simulink library "powerlib_models"  (Simulink 6.0)
settings: Solver=ode45  SolverMode=SingleTasking  StartTime=0.0  StopTime=10.0  RelTol=1e-3
values from neighbouring files (symbols this model uses):
  Ts = get(handles.edit1,'string')    [powergui.m]
undefined symbols (not defined in the file or in its folder): A, a0, a1, a2, a3, a4, a5, Ac, Amplitude, Amplitudes, B, BaseCurrent, BaseFlux, Bc, C, Capacitance, Cc, Columns, ConnectionType, Cs, ctrl, current, Current, damp, Dc, Dd, DiscIntNeverNeededParam, dref, dwo, exc, excAxis, F, Flux, fnom, Frequency, FreqVps, Gain1, gate, GH, GHd, GI, GId, GL, GLd, H, HarmonicGeneration, HT, hyd, I1_init, ib, ib2, Id1o, Inductance, InitialFlux, InitialSlope, io, Iq1o, isfinite, j, J ... (+138)
libraries: powerlib_models x32, powerlib_extras x4
(part 7 of 11)

== system powerlib_models/Discrete/3_Phase_Prog_Source/Harmonic A generation ==
  Enable : Inport  Port=1  LatchInput=off
  Gain2 : Gain  Gain=2*pi*n_Harmo  SaturateOnIntegerOverflow=on
  Gain3 : Gain  Gain=pi/180  SaturateOnIntegerOverflow=on
  Multiport Switch : MultiPortSwitch  Inputs=3  InputSameDT=on
  Negative-sequence : Constant  Value=[0 2*pi/3 -2*pi/3]
  Phase_Harmo : Constant  Value=Phase_Harmo
  Phase_Harmo1 : Constant  Value=Mag_Harmo
  Phase_Harmo2 : Constant  Value=Seq_Harmo
  Positive-sequence : Constant  Value=[0 -2*pi/3 2*pi/3]
  Product : Product  SaturateOnIntegerOverflow=on  InputSameDT=on
  Product1 : Product  Inputs=3  SaturateOnIntegerOverflow=on  InputSameDT=on
  Sum : Sum  Inputs=+++  SaturateOnIntegerOverflow=on  InputSameDT=on
  Sum1 : Sum  SaturateOnIntegerOverflow=on  InputSameDT=on
  Trigonometric Function1 : Trigonometry
  Zero-sequence : Constant  Value=[0 0 0]
  t : DigitalClock  SampleTime=Ts
  valp_nom1 : Constant  Value=Freq_Vps
  valp_nom2 : Constant
  HarmoA : Outport
  wires:
  Gain3/1 -> Sum/2
  Phase_Harmo/1 -> Gain3/1
  Enable/1 -> Product1/1
  valp_nom2/1 -> Sum1/2
  Phase_Harmo2/1 -> Sum1/1
  Sum1/1 -> Multiport Switch/1
  Phase_Harmo1/1 -> Product1/2
  Product1/1 -> HarmoA/1
  Trigonometric Function1/1 -> Product1/3
  Product/1 -> Sum/1
  t/1 -> Product/1
  Gain2/1 -> Product/2
  valp_nom1/1 -> Gain2/1
  Negative-sequence/1 -> Multiport Switch/4
  Positive-sequence/1 -> Multiport Switch/3
  Zero-sequence/1 -> Multiport Switch/2
  Multiport Switch/1 -> Sum/3
  Sum/1 -> Trigonometric Function1/1

== system powerlib_models/Discrete/3_Phase_Prog_Source/Harmonic B generation ==
  Enable : Inport  Port=1  LatchInput=off
  Gain2 : Gain  Gain=2*pi*n_Harmo  SaturateOnIntegerOverflow=on
  Gain3 : Gain  Gain=pi/180  SaturateOnIntegerOverflow=on
  Multiport Switch : MultiPortSwitch  Inputs=3  InputSameDT=on
  Negative-sequence : Constant  Value=[0 2*pi/3 -2*pi/3]
  Phase_Harmo : Constant  Value=Phase_Harmo
  Phase_Harmo1 : Constant  Value=Mag_Harmo
  Phase_Harmo2 : Constant  Value=Seq_Harmo
  Positive-sequence : Constant  Value=[0 -2*pi/3 2*pi/3]
  Product : Product  SaturateOnIntegerOverflow=on  InputSameDT=on
  Product1 : Product  Inputs=3  SaturateOnIntegerOverflow=on  InputSameDT=on
  Sum : Sum  Inputs=+++  SaturateOnIntegerOverflow=on  InputSameDT=on
  Sum1 : Sum  SaturateOnIntegerOverflow=on  InputSameDT=on
  Trigonometric Function1 : Trigonometry
  Zero-sequence : Constant  Value=[0 0 0]
  t : DigitalClock  SampleTime=Ts
  valp_nom1 : Constant  Value=Freq_Vps
  valp_nom2 : Constant
  HarmoB : Outport
  wires:
  Gain3/1 -> Sum/2
  Phase_Harmo/1 -> Gain3/1
  Sum/1 -> Trigonometric Function1/1
  Multiport Switch/1 -> Sum/3
  Zero-sequence/1 -> Multiport Switch/2
  Positive-sequence/1 -> Multiport Switch/3
  Negative-sequence/1 -> Multiport Switch/4
  valp_nom1/1 -> Gain2/1
  Gain2/1 -> Product/2
  t/1 -> Product/1
  Product/1 -> Sum/1
  Trigonometric Function1/1 -> Product1/3
  Product1/1 -> HarmoB/1
  Phase_Harmo1/1 -> Product1/2
  Sum1/1 -> Multiport Switch/1
  Phase_Harmo2/1 -> Sum1/1
  valp_nom2/1 -> Sum1/2
  Enable/1 -> Product1/1

== system powerlib_models/Discrete/3_Phase_Prog_Source/Timer ==
  Clock : Clock
  Look-Up Table : Lookup  DialogController=Simulink.DDGSource  InputValues=tv  OutputValues=opv  SaturateOnIntegerOverflow=on
  Out : Outport
  wires:
  Look-Up Table/1 -> Out/1
  Clock/1 -> Look-Up Table/1

== system powerlib_models/Discrete/3_Phase_Prog_Source/Variation SubSystem ==
  VariationType : Inport  Port=1  LatchInput=off
  Constant : Constant  Value=2
  Constant1 : Constant  Value=0
  Constant2 : Constant
  Constant3 : Constant
  Constant4 : Constant  Value=0
  Constant5 : Constant  Value=0
  Data Type  Conversion1 : DataTypeConversion  OutDataTypeMode=boolean  SaturateOnIntegerOverflow=on  RndMeth=Zero
  Data Type  Conversion2 : DataTypeConversion  Orientation=up  OutDataTypeMode=boolean  SaturateOnIntegerOverflow=on  RndMeth=Zero
  Discrete-Time Integrator1 : DiscreteIntegrator  SampleTime=Ts  ICPrevOutput=DiscIntNeverNeededParam  ICPrevScaledInput=DiscIntNeverNeededParam
  Gain1 : Gain  Gain=2*pi  SaturateOnIntegerOverflow=on
  Logical Operator : Logic
  Logical Operator1 : Logic  Orientation=up  Operator=NOT
  Multiport Switch1 : MultiPortSwitch  InputSameDT=on
  Product : Product  SaturateOnIntegerOverflow=on  InputSameDT=on
  Product1 : Product  SaturateOnIntegerOverflow=on  InputSameDT=on
  Product2 : Product  SaturateOnIntegerOverflow=on  InputSameDT=on
  Relational Operator : RelationalOperator  Operator===  InputSameDT=on
  Relational Operator1 : RelationalOperator  Operator===  InputSameDT=on
  Step : Step  Time=Ton_Variation  SampleTime=Ts
  Step1 : Step  Time=Toff_Variation  Before=1  After=0  SampleTime=Ts
  Switch{,1..3} (4 alike) : Switch  Threshold=0.5  InputSameDT=on
  Trigonometric Function1 : Trigonometry
  Unit Delay : UnitDelay  Orientation=left  SampleTime=Ts
  valp_nom6 : Constant  Value=VariationStep
  valp_nom7 : Constant  Value=VariationRate
  valp_nom8 : Constant  Value=VariationMag
  valp_nom9 : Constant  Value=VariationFreq
  Value : Outport
  wires:
  Data Type  Conversion1/1 -> Logical Operator/2
  Constant5/1 -> Multiport Switch1/5
  Logical Operator1/1 -> Logical Operator/1
  Logical Operator/1 -> Switch3/2
  Step1/1 -> Switch2/2, Data Type  Conversion2/1  "Toff"
  Constant3/1 -> Relational Operator1/2
  Switch3/1 -> Value/1
  Switch2/1 -> Switch3/3, Unit Delay/1
  Constant1/1 -> Switch3/1
  Unit Delay/1 -> Switch2/3
  Multiport Switch1/1 -> Switch2/1
  Step/1 -> Product2/2, Switch/2  "Ton"
  VariationType/1 -> Relational Operator/1, Relational Operator1/1, Multiport Switch1/1
  Discrete-Time Integrator1/1 -> Multiport Switch1/3, Product1/1  "Ramp"
  Product2/1 -> Multiport Switch1/2  "Step"
  valp_nom6/1 -> Product2/1
  Relational Operator/1 -> Switch1/2
  Switch/1 -> Discrete-Time Integrator1/1
  Constant/1 -> Relational Operator/2
  Switch1/1 -> Switch/1
  Constant4/1 -> Switch/3
  Constant2/1 -> Switch1/3
  valp_nom7/1 -> Switch1/1
  Product/1 -> Multiport Switch1/4  "Mod"
  Product1/1 -> Trigonometric Function1/1
  Gain1/1 -> Product1/2
  valp_nom9/1 -> Gain1/1
  valp_nom8/1 -> Product/1
  Trigonometric Function1/1 -> Product/2
  Data Type  Conversion2/1 -> Logical Operator1/1
  Relational Operator1/1 -> Data Type  Conversion1/1

== system powerlib_models/Discrete/Dynamic_Load/Discrete 3-phase PLL ==
  note: Pierre Giroux, Gilbert Sybille
      | Power System Laboratory, IREQ
      | Hydro-Quebec
  note: Discrete 3-phase PLL
  note: link disabled
  note: link disabled
  note: link disabled
  note: link disabled
  note: link broken
  Vab_bc (pu) : Inport  Port=1  PortDimensions=2  LatchInput=off
  Constant4 : Constant  Value=2*pi
  Discrete PI Controller : Subsystem  AncestorBlock=|  mask(Discrete PI Controller){Kp=Kp, Ki=Ki, Par_Limits=2*pi*Finit*[1.25 0.75], Init=2*pi*Finit, Ts=Ts}
      | powerlib_extras/Discrete 
      | Control Blocks/Discrete
      | PI Controller
      mask prompts: Kp "Proportional gain (Kp):"; Ki "Integral gain (Ki):"; Par_Limits "Output limits: [ Upper   Lower ]"; Init "Output initial value:"; Ts "Sample time:"
      mask help: This block implements a discrete PI controller.
      mask init:
      | UpperLimit=Par_Limits(1);
      | LowerLimit=Par_Limits(2);
      mask Display: disp('PI');
  Discrete Rate Limiter : Subsystem  AncestorBlock=|  mask{R=10, F=-10, Vinit=Finit, Ts=Ts}
      | powerlib_extras/Discrete 
      | Control Blocks/Discrete
      | Rate Limiter
      mask prompts: R "Rising slew rate:"; F "Falling slew rate:"; Vinit "Initial input:"; Ts "Sample time:"
      mask help: DISCRETE BLOCK : Limit rising and falling rates of signal
      mask init:
      | UpperLimit=R*Ts;
      | LowerLimit=F*Ts;
      mask Display: disp('Discrete\nRate\nLimiter')
  Discrete Variable Frequency Mean value : Subsystem  AncestorBlock=|  mask(Discrete Variable-Frequency Mean Value){Finit=Finit, Fmin=45, Vinit=0, Ts=Ts}
      | powerlib_extras/Discrete
      | Measurements/Discrete
      | Variable Frequency
      | Mean value
      mask prompts: Finit "Initial frequency (Hz):"; Fmin "Minimum frequency (Hz):"; Vinit "Initial input (DC component):"; Ts "Sample time:"
      mask help:
      | This discrete block computes the mean value of the input signal (port In) over a running window of one cycle of a specified frequency (port Freq).
      |
      | For the first cycle of simulation (specified by the parameter "Initial frequency"), the ouput is held to the value of the  "Initial input" parameter.
      |
      | The value of the parameter "Minimum frequency" is used to determine the buffer size of the "Variable Transport Delay" block found inside this subsystem.
      mask init:
      | MaxDelay=1/Fmin+Ts;
  Discrete  2nd-Order Filter : Subsystem  AncestorBlock=|  mask(Discrete 2nd-Order Filter){FilterType=Lowpass, Fo=25, Zeta=0.707, Ts=Ts, Initialize=on, Vac_Init=[0 0 Finit], Vdc_Init=Finit, PlotResponse=off, param1=[1 500 0.1]}
      | powerlib_extras/Discrete 
      | Control Blocks/Discrete 
      | 2nd-Order
      | Filter
      mask prompts: FilterType "Filter Type:"; Fo "Cut-off frequency (Hz):"; Zeta "Damping factor Zeta ( Q = 1 / (2*Zeta) ):"; Ts "Sample time:"; Initialize "Initialize filter states"; Vac_Init "AC initial input: [ Mag  Phase(degrees)  Freq(Hz) ]"; Vdc_Init "DC Initial input:"; PlotResponse "Plot filter response"; param1 "Frequency range(Hz) : [Start  End  Inc.]"
      mask init:
      | Wo=2*pi*Fo;
      | str=sprintf(' Fo=%iHz\n\n',Fo);
      | switch FilterType
      | case 1, % Lowpass
      |        X=[0 1 2 3 4];
      |        Y=[-2 -2 -3 -4 -4];
      |        n2=0;n1=0;n0=Wo*Wo;
      |        d2=1;d1=2*Zeta*Wo;d0=Wo*Wo;
      |  case 2,   % Highpass
      |        X=[0 1 2 3 4];
      |        Y=[-4 -4 -3 -2 -2];
      |        n2=1;n1=0;n0=0;
      |        d2=1;d1=2*Zeta*Wo;d0=Wo*Wo;
      |     case 3,   % Bandpass
      |        X=[0 1 2 3 4 5 ];
      |        Y=[-3 -3 -2 -2 -3 -3];
      |        n2=0;n1=2*Zeta*Wo;n0=0;
      |        d2=1;d1=2*Zeta*Wo;d0=Wo*Wo;
      |     case 4,  %Bandstop (Notch)
      |        X=[0 1 2 3 4 5 ];
      |        Y=[-2 -2 -3 -3 -2 -2];
      |        n2=1;n1=0;n0=Wo*Wo;
      |        d2=1;d1=2*Zeta*Wo;d0=Wo*Wo;
      |     end
      | %
      | numc=[n2 n1 n0];
      | denc=[d2 d1 d0];
      | [Ac,Bc,Cc,Dc]=tf2ss(numc,denc);
      | %
      | %  Conversion to discrete transfer function
      | nstates = size(Ac,1);
      | invexp = inv(eye(nstates) - (Ts/2)*Ac);
      | Ad = invexp*(eye(nstates) + (Ts/2)*Ac);
      | Bd = invexp*Bc;
      | Cd = Cc*invexp*Ts;
      | Dd = Cc*invexp*Bc*(Ts/2) + Dc;
      | %
      | if Initialize==1  % Compute initial conditions on states
      | u1=Vac_Init(1)*exp(j*Vac_Init(2)*pi/180);
      | u2=Vdc_Init*exp(j*90*pi/180);
      | u=u1+u2;
      | u0=imag(u); % input at  t=0;
      | I=eye(size(Ac));
      | sI1=I*j*(2*pi*Vac_Init(3));
      | sI2=I*j*0;
      | x=inv(sI1-Ac)*Bc*u1 + inv(sI2-Ac)*Bc*u2;
      | x0c=imag(x);
      | x0d=(I-Ac*Ts/2)*x0c/Ts - Bc/2*u0;
      | else
      | x0d=0;
      | end
      | %
      | if PlotResponse==1 % Plot frequency and step response
      | figure(1)
      | sys=ss(Ad,Bd,Cd,Dd,Ts);
      | f=param1(1):param1(3):param1(2);
      | w=2*pi*f;
      | [mag phase]=bode(sys,w);
      | subplot(2,1,1)
      | plot(f,squeeze(mag))
      | title('Magnitude')
      | grid
      | subplot(2,1,2)
      | plot(f,squeeze(phase))
      | title('Phase (degrees)')
      | xlabel('Hz')
      | grid
      | figure(2)
      | step(sys)
      | end
      mask StyleString: popup(Lowpass|Highpass|Bandpass|Bandstop (Notch)),edit,edit,edit,checkbox,edit,edit,checkbox,edit
      mask CallbackString: ||||p5=get_param(gcb,'Initialize');if strcmp(p5,'on');visible={'on','on','on','on','on','on','on','on',get_param(gcb,'PlotResponse')};else;visible={'on','on','on','on','on','off','off','on',get_param(gcb,'PlotResponse')};end;set_param(gcb,'MaskVisibilities',visible)|||p8=get_param(gcb,'PlotResponse');if strcmp(p8,'on');visible={'on','on','on','on','on',get_param(gcb,'Initialize'),get_param(gcb,'Initialize'),'on','on'};else;visible={'on','on','on','on','on',get_param(gcb,'Initialize'),get_param(gcb,'Initialize'),'on','off'};end;set_param(gcb,'MaskVisibilities',visible)|
      mask Display:
      | plot(X,Y);
      | disp(str);
  Discrete-Time Integrator : DiscreteIntegrator  InitialCondition=Phase_Init*pi/180  SampleTime=Ts  ICPrevOutput=DiscIntNeverNeededParam  ICPrevScaledInput=DiscIntNeverNeededParam
  Gain10 : Gain  Gain=1/2/pi  SaturateOnIntegerOverflow=on
  Math Function : Math  Operator=mod  SaturateOnIntegerOverflow=on
  Mux2 : Mux  Inputs=2
  Trigonometric Function : Trigonometry
  Trigonometric Function2 : Trigonometry  Operator=cos
  Unit Delay : UnitDelay  X0=Finit  SampleTime=Ts
  abc_to_dq1 : Subsystem
  Freq : Outport
  Vd : Outport  Port=2
  Vq : Outport  Port=3
  sin_cos : Outport  Port=4
  wires:
  Discrete  2nd-Order Filter/1(Out) -> Unit Delay/1
  Unit Delay/1 -> Discrete Variable Frequency Mean value/1(Freq), Freq/1
  Discrete Rate Limiter/1(Out) -> Discrete  2nd-Order Filter/1(In)
  Gain10/1 -> Discrete Rate Limiter/1(In)
  Discrete PI Controller/1(Out) -> Gain10/1, Discrete-Time Integrator/1  "W"
  Mux2/1 -> sin_cos/1, abc_to_dq1/2(sin_cos)
  Trigonometric Function2/1 -> Mux2/2
  Trigonometric Function/1 -> Mux2/1
  Math Function/1 -> Trigonometric Function2/1, Trigonometric Function/1
  Discrete-Time Integrator/1 -> Math Function/1
  Constant4/1 -> Math Function/2
  abc_to_dq1/2(vq) -> Discrete Variable Frequency Mean value/2(In), Vq/1  "Vq"
  Vab_bc (pu)/1 -> abc_to_dq1/1(Vab_bc)
  Discrete Variable Frequency Mean value/1(Mean) -> Discrete PI Controller/1(Error)
  abc_to_dq1/1(vd) -> Vd/1

== system powerlib_models/Discrete/Dynamic_Load/Positive Sequence  current ==
  note: kp=Vmin^(np-2)/Vo^np
      | kq=Vmin^(nq-2)/Vo^nq
  note: V<Vmin
      | Constant impedance load :
      |  P=Po*kp*V^2
      | Q=Qo*kq*V^2
  note: V>Vmin :
      |
      |    P=Po*(V/Vo)^np
      |    Q=Qo*(V/Vo)^np
  note: I1= (S/V1)'
  note: link disabled
  note: link disabled
  V1(pu) : Inport  Port=1  PortDimensions=1  LatchInput=off
  S_ext : Inport  Port=2  PortDimensions=1  LatchInput=off
  Complex to Magnitude-Angle : ComplexToMagnitudeAngle  Output=Magnitude
  Complex to Real-Imag1 : ComplexToRealImag
  Conj1 : Math  Operator=conj  SaturateOnIntegerOverflow=on
  Math Function : Math  Operator=square  SaturateOnIntegerOverflow=on
  Mux1 : Mux  Inputs=3
  Mux2 : Mux  Inputs=2
  Mux3 : Mux  Inputs=2
  P0/ (Vo^np) : Gain  Gain=P0/(Mag_V0^np)  SaturateOnIntegerOverflow=on
  PQ_ext : Constant  Value=PQext
  Product : Product  Inputs=/*  SaturateOnIntegerOverflow=on  InputSameDT=on
  Q0/(Vo^nq) : Gain  Gain=Q0/(Mag_V0^nq)  SaturateOnIntegerOverflow=on
  Real-Imag to Complex : RealImagToComplex
  Switch1 : Switch  Threshold=0.5  InputSameDT=on
  Switch3 : Switch  Threshold=Vmin  InputSameDT=on
  Switch4 : Switch  Threshold=Vmin  InputSameDT=on
  TF_P : Subsystem  AncestorBlock=|  mask(Discrete Lead-Lag Controller){T1=Tp1, T2=Tp2, V_Init=P0, Ts=Ts}
      | powerlib_extras/Discrete 
      | Control Blocks/Discrete
      | Lead-Lag
      mask prompts: T1 "Time constant T1 (s):"; T2 "Time constant T2 (s):"; V_Init "Initial input and output:"; Ts "Sample time (s):"
      mask help:
      | This block implements a discrete lead-lag controller:
      |
      |          1+T1s
      | H(s)= ------
      |          1+T2s
      |
      | States are initialized according to initial input anf output value so that simulation starts in steady state.
      mask init: same as powerlib_models/Discrete/Excitation_System/Lead Lag Compensator tc.s+1 / tb.s+1
      mask Display: disp('1+T1s\n---\n1+T2s')
  TF_Q : Subsystem  AncestorBlock=|  mask(Discrete Lead-Lag Controller){T1=Tq1, T2=Tq2, V_Init=Q0, Ts=Ts}
      | powerlib_extras/Discrete 
      | Control Blocks/Discrete
      | Lead-Lag
      mask prompts: T1 "Time constant T1 (s):"; T2 "Time constant T2 (s):"; V_Init "Initial input and output:"; Ts "Sample time (s):"
      mask help:
      | This block implements a discrete lead-lag controller:
      |
      |          1+T1s
      | H(s)= ------
      |          1+T2s
      |
      | States are initialized according to initial input anf output value so that simulation starts in steady state.
      mask init: same as powerlib_models/Discrete/Excitation_System/Lead Lag Compensator tc.s+1 / tb.s+1
      mask Display: disp('1+T1s\n---\n1+T2s')
  V^nq : Fcn  Expr=u[1]^u[2]
  V^nq , : Fcn  Expr=u[1]^u[2]
  Vmin^(np-2) : Gain  Gain=Vmin^(np-2)  SaturateOnIntegerOverflow=on
  Vmin^(nq-2) : Gain  Gain=Vmin^(nq-2)  SaturateOnIntegerOverflow=on
  np : Constant  Value=np
  nq : Constant  Value=nq
  pu>V : Gain  Gain=Vnom*sqrt(3)/sqrt(2)  SaturateOnIntegerOverflow=on
  I1(A) : Outport
  VPQ : Outport  Port=2
  wires:
  Vmin^(nq-2)/1 -> Switch4/3
  V^nq ,/1 -> Switch3/1
  Vmin^(np-2)/1 -> Switch3/3
  Math Function/1 -> Vmin^(nq-2)/1, Vmin^(np-2)/1
  V^nq/1 -> Switch4/1
  V1(pu)/1 -> Complex to Magnitude-Angle/1, pu>V/1
  Mux3/1 -> V^nq/1
  nq/1 -> Mux3/2
  Mux2/1 -> V^nq ,/1
  np/1 -> Mux2/2
  Switch3/1 -> P0/ (Vo^np)/1
  Q0/(Vo^nq)/1 -> TF_Q/1(In1)
  P0/ (Vo^np)/1 -> TF_P/1(In1)
  Switch4/1 -> Q0/(Vo^nq)/1
  Product/1 -> Conj1/1
  Conj1/1 -> I1(A)/1
  Switch1/1 -> Product/2, Complex to Real-Imag1/1  "S=P+jQ"
  Real-Imag to Complex/1 -> Switch1/3  "S_dyn"
  S_ext/1 -> Switch1/1
  PQ_ext/1 -> Switch1/2
  pu>V/1 -> Product/1
  Complex to Magnitude-Angle/1 -> Math Function/1, Mux3/1, Mux2/1, Switch3/2, Switch4/2, Mux1/1
  Mux1/1 -> VPQ/1
  Complex to Real-Imag1/1 -> Mux1/2
  Complex to Real-Imag1/2 -> Mux1/3
  TF_P/1(Out1) -> Real-Imag to Complex/1
  TF_Q/1(Out1) -> Real-Imag to Complex/2

== system powerlib_models/Discrete/Excitation_System/Damping kf.s / (tf.s +1) ==
  note: link disabled
  In : Inport  Orientation=left  Port=1  LatchInput=off
  1st-Order Discrete Filter : Subsystem  Orientation=left  AncestorBlock=|  mask(Discrete 1st-Order Filter){FilterType=Highpass, Tc=tf, Ts=Ts, Initialize=on, Vac_Init=[0 0 60], Vdc_Init=kf*v0(2)/tf, PlotResponse=off, param1=[1 500 0.1]}
      | powerlib_extras/Discrete 
      | Control Blocks/Discrete
      | 1st-Order
      | Discrete Filter
      mask prompts: FilterType "Filter Type:"; Tc "Time constant (s):"; Ts "Sample time:"; Initialize "Initialize filter states"; Vac_Init "AC initial input: [ Mag  Phase(degrees)  Freq(Hz) ]"; Vdc_Init "DC Initial input:"; PlotResponse "Plot filter response"; param1 "Frequency range(Hz) : [Start  End  Inc.]"
      mask init: same as powerlib_models/Discrete/Excitation_System/Low Pass Filter 1 / (tr.s +1) (with IC)
      mask StyleString: popup(Lowpass|Highpass),edit,edit,checkbox,edit,edit,checkbox,edit
      mask CallbackString: |||p4=get_param(gcb,'Initialize');if strcmp(p4,'on');visible={'on','on','on','on','on','on','on',get_param(gcb,'PlotResponse')};else;visible={'on','on','on','on','off','off','on',get_param(gcb,'PlotResponse')};end;set_param(gcb,'MaskVisibilities',visible)|||p7=get_param(gcb,'PlotResponse');if strcmp(p7,'on');visible={'on','on','on','on',get_param(gcb,'Initialize'),get_param(gcb,'Initialize'),'on','on'};else;visible={'on','on','on','on',get_param(gcb,'Initialize'),get_param(gcb,'Initialize'),'on','off'};end;set_param(gcb,'MaskVisibilities',visible)|
      mask Display: plot(X,Y);
  Gain : Gain  Orientation=left  Gain=kf/tf  SaturateOnIntegerOverflow=on
  Out : Outport  Orientation=left
  wires:
  1st-Order Discrete Filter/1(Out) -> Out/1
  Gain/1 -> 1st-Order Discrete Filter/1(In)
  In/1 -> Gain/1

== system powerlib_models/Discrete/Excitation_System/Exciter  1 / (te.s + ke) ==
  note: link disabled
  In : Inport  Port=1  LatchInput=off
  1st order Lowpass : Subsystem  AncestorBlock=|  mask(Discrete 1st-Order Filter){FilterType=Lowpass, Tc=te/ke, Ts=Ts, Initialize=on, Vac_Init=[0.0 0 60], Vdc_Init=v0(2), PlotResponse=off, param1=[1 500 0.1]}
      | powerlib_extras/Discrete 
      | Control Blocks/Discrete
      | 1st-Order
      | Discrete Filter
      mask prompts: FilterType "Filter Type:"; Tc "Time constant (s):"; Ts "Sample time:"; Initialize "Initialize filter states"; Vac_Init "AC initial input: [ Mag  Phase(degrees)  Freq(Hz) ]"; Vdc_Init "DC Initial input:"; PlotResponse "Plot filter response"; param1 "Frequency range(Hz) : [Start  End  Inc.]"
      mask init: same as powerlib_models/Discrete/Excitation_System/Low Pass Filter 1 / (tr.s +1) (with IC)
      mask StyleString: popup(Lowpass|Highpass),edit,edit,checkbox,edit,edit,checkbox,edit
      mask CallbackString: |||p4=get_param(gcb,'Initialize');if strcmp(p4,'on');visible={'on','on','on','on','on','on','on',get_param(gcb,'PlotResponse')};else;visible={'on','on','on','on','off','off','on',get_param(gcb,'PlotResponse')};end;set_param(gcb,'MaskVisibilities',visible)|||p7=get_param(gcb,'PlotResponse');if strcmp(p7,'on');visible={'on','on','on','on',get_param(gcb,'Initialize'),get_param(gcb,'Initialize'),'on','on'};else;visible={'on','on','on','on',get_param(gcb,'Initialize'),get_param(gcb,'Initialize'),'on','off'};end;set_param(gcb,'MaskVisibilities',visible)|
      mask Display: plot(X,Y);
  Gain : Gain  Gain=1/ke  SaturateOnIntegerOverflow=on
  Out : Outport
  wires:
  Gain/1 -> 1st order Lowpass/1(In)
  In/1 -> Gain/1
  1st order Lowpass/1(Out) -> Out/1

== system powerlib_models/Discrete/Excitation_System/Lead Lag Compensator tc.s+1 / tb.s+1 ==
  In1 : Inport  Port=1  LatchInput=off
  Discrete State-Space : DiscreteStateSpace  A=Ad  B=Bd  C=Cd  D=Dd  X0=x0d  SampleTime=Ts
  Out1 : Outport
  wires:
  In1/1 -> Discrete State-Space/1
  Discrete State-Space/1 -> Out1/1

== system powerlib_models/Discrete/Excitation_System/Low Pass Filter 1 / (tr.s +1) (with IC) ==
  In : Inport  Port=1  LatchInput=off
  Discrete State-Space : DiscreteStateSpace  A=Ad  B=Bd  C=Cd  D=Dd  X0=x0d  SampleTime=Ts
  Out : Outport  InitialOutput=0
  wires:
  In/1 -> Discrete State-Space/1
  Discrete State-Space/1 -> Out/1

== system powerlib_models/Discrete/Excitation_System/Main Regulator ka / (ta.s +1) ==
  note: link disabled
  In : Inport  Port=1  LatchInput=off
  1st order Lowpass : Subsystem  AncestorBlock=|  mask(Discrete 1st-Order Filter){FilterType=Lowpass, Tc=ta, Ts=Ts, Initialize=on, Vac_Init=[0.0 0 60], Vdc_Init=ke*v0(2), PlotResponse=off, param1=[1 500 0.1]}
      | powerlib_extras/Discrete 
      | Control Blocks/Discrete
      | 1st-Order
      | Discrete Filter
      mask prompts: FilterType "Filter Type:"; Tc "Time constant (s):"; Ts "Sample time:"; Initialize "Initialize filter states"; Vac_Init "AC initial input: [ Mag  Phase(degrees)  Freq(Hz) ]"; Vdc_Init "DC Initial input:"; PlotResponse "Plot filter response"; param1 "Frequency range(Hz) : [Start  End  Inc.]"
      mask init: same as powerlib_models/Discrete/Excitation_System/Low Pass Filter 1 / (tr.s +1) (with IC)
      mask StyleString: popup(Lowpass|Highpass),edit,edit,checkbox,edit,edit,checkbox,edit
      mask CallbackString: |||p4=get_param(gcb,'Initialize');if strcmp(p4,'on');visible={'on','on','on','on','on','on','on',get_param(gcb,'PlotResponse')};else;visible={'on','on','on','on','off','off','on',get_param(gcb,'PlotResponse')};end;set_param(gcb,'MaskVisibilities',visible)|||p7=get_param(gcb,'PlotResponse');if strcmp(p7,'on');visible={'on','on','on','on',get_param(gcb,'Initialize'),get_param(gcb,'Initialize'),'on','on'};else;visible={'on','on','on','on',get_param(gcb,'Initialize'),get_param(gcb,'Initialize'),'on','off'};end;set_param(gcb,'MaskVisibilities',visible)|
      mask Display: plot(X,Y);
  Gain : Gain  Gain=ka  SaturateOnIntegerOverflow=on
  Out : Outport
  wires:
  1st order Lowpass/1(Out) -> Out/1
  In/1 -> Gain/1
  Gain/1 -> 1st order Lowpass/1(In)

== system powerlib_models/Discrete/Excitation_System/proportionnal saturation ==
  Efd : Inport  Port=1  LatchInput=off
  Vtf : Inport  Port=2  LatchInput=off
  Constant : Constant  Value=kp
  Constant1 : Constant  Value=efmin
  Constant3 : Constant  Value=0
  Data Type  Conversion{,1..3} (4 alike) : DataTypeConversion  OutDataTypeMode=double  SaturateOnIntegerOverflow=on  RndMeth=Zero
  Logical Operator : Logic
  Logical Operator1 : Logic  Operator=NOT  Inputs=1
  Logical Operator2 : Logic  Operator=NOT  Inputs=1
  Product : Product  SaturateOnIntegerOverflow=on  InputSameDT=on
  Product1 : Product  SaturateOnIntegerOverflow=on  InputSameDT=on
  Product2 : Product  SaturateOnIntegerOverflow=on  InputSameDT=on
  Relational Operator : RelationalOperator  Operator===  InputSameDT=on
  Relational Operator1 : RelationalOperator  Operator=<  InputSameDT=on
  Relational Operator2 : RelationalOperator  Operator=>  InputSameDT=on
  Sum : Sum  SaturateOnIntegerOverflow=on  InputSameDT=on
  Sum1 : Sum  Inputs=+++  SaturateOnIntegerOverflow=on  InputSameDT=on
  Vfdmax : Gain  Gain=efmax  SaturateOnIntegerOverflow=on
  Vfdmax1 : Gain  Gain=kp  SaturateOnIntegerOverflow=on
  Ef : Outport  InitialOutput=0
  wires:
  Data Type  Conversion3/1 -> Vfdmax/1
  Relational Operator/1 -> Data Type  Conversion3/1
  Data Type  Conversion2/1 -> Product2/1
  Logical Operator2/1 -> Data Type  Conversion2/1
  Data Type  Conversion1/1 -> Product1/2
  Logical Operator1/1 -> Data Type  Conversion1/1
  Data Type  Conversion/1 -> Product/2
  Logical Operator/1 -> Data Type  Conversion/1
  Product1/1 -> Sum1/2
  Product2/1 -> Sum1/3
  Product/1 -> Sum1/1
  Sum1/1 -> Ef/1
  Efd/1 -> Product/1, Relational Operator1/1, Relational Operator2/1
  Constant1/1 -> Product1/1, Relational Operator2/2
  Relational Operator1/1 -> Logical Operator/2, Logical Operator2/1
  Relational Operator2/1 -> Logical Operator/1, Logical Operator1/1
  Sum/1 -> Relational Operator1/2, Product2/2
  Vfdmax1/1 -> Sum/1
  Vfdmax/1 -> Sum/2
  Constant3/1 -> Relational Operator/2
  Constant/1 -> Relational Operator/1
  Vtf/1 -> Vfdmax1/1

== system powerlib_models/Discrete/GTO-IGBT Bridge/Diode Logic ==
  note: Note : Block D1 (D2) if D2 (D1) is triggered.
      |  Diodes always trigerred, even with capacitive snubbers.
  Vak : Inport  Port=1  LatchInput=off
  Ipos : Inport  Port=2  LatchInput=off
  G : Inport  Port=3  LatchInput=off
  0 2 : Constant  Value=0
  0 3 : Constant
  1 : Logic
  2 : Logic  Operator=OR
  3 : Logic  Operator=OR
  Block D : Selector  Orientation=up  Elements=Selec_Diode  InputPortWidth=nb_switch
  Blocking Diodes : Subsystem
  Data Type  Conversion5 : DataTypeConversion  OutDataTypeMode=boolean  SaturateOnIntegerOverflow=on  RndMeth=Zero
  Logical Operator3 : Logic  Operator=NOT
  Trig.  Diodes : Subsystem  TreatAsAtomicUnit=on
  b6 : RelationalOperator  Operator=>  InputSameDT=on
  status : Outport  InitialOutput=0
  wires:
  Block D/1 -> 3/2
  3/1 -> Logical Operator3/1
  2/1 -> status/1
  1/1 -> 2/1
  Logical Operator3/1 -> 1/2
  Trig.  Diodes/1(Trig D) -> Block D/1, 2/2
  Blocking Diodes/1(Block.D) -> 3/1
  0 3/1 -> Trig.  Diodes/Enable
  Ipos/1 -> Trig.  Diodes/2(Ipos)
  G/1 -> Trig.  Diodes/1(G), Blocking Diodes/1(G)
  0 2/1 -> b6/2
  Vak/1 -> b6/1
  b6/1 -> Data Type  Conversion5/1
  Data Type  Conversion5/1 -> 1/1

== system powerlib_models/Discrete/GTO-IGBT Bridge/GTO Logic ==
  Vak : Inport  Port=1  LatchInput=off
  G : Inport  Port=2  LatchInput=off
  " " : RelationalOperator  Operator=>  InputSameDT=on
  "    " : Constant  Value=0
  ". " : Logic
  Data Type  Conversion1 : DataTypeConversion  OutDataTypeMode=boolean  SaturateOnIntegerOverflow=on  RndMeth=Zero
  Data Type  Conversion2 : DataTypeConversion  OutDataTypeMode=boolean  SaturateOnIntegerOverflow=on  RndMeth=Zero
  Data Type  Conversion3 : DataTypeConversion  OutDataTypeMode=boolean  SaturateOnIntegerOverflow=on  RndMeth=Zero
  Vpos : Constant  Value=0
  b : RelationalOperator  Operator=>  InputSameDT=on
  status : Outport  InitialOutput=0
  wires:
  ". "/1 -> status/1
  Vak/1 -> b/1
  Vpos/1 -> b/2
  G/1 -> " "/1
  b/1 -> Data Type  Conversion1/1
  Data Type  Conversion1/1 -> ". "/1
  " "/1 -> Data Type  Conversion2/1
  Data Type  Conversion2/1 -> ". "/2
  "    "/1 -> Data Type  Conversion3/1
  Data Type  Conversion3/1 -> " "/2

== system powerlib_models/Discrete/GTO-IGBT Bridge/Tail discrete ==
  Iak : Inport  Port=1  LatchInput=off
  switch : Inport  Port=2  LatchInput=off
  Enable : EnablePort  StatesWhenEnabling=reset
  1 : Constant
  Discrete-Time Integrator : DiscreteIntegrator  IntegratorMethod=Integration: Trapezoidal  ExternalReset=falling  SampleTime=Ts  ICPrevOutput=DiscIntNeverNeededParam  ICPrevScaledInput=DiscIntNeverNeededParam
  Look-Up Table : Lookup  DialogController=Simulink.DDGSource  InputValues="[  0    Tf+eps Tf+Tt+2*eps  Tf+Tt+3*eps ]"  OutputValues="[  1    0.1*(Tt>0) 0 0]"  SaturateOnIntegerOverflow=on
  Product : Product  SaturateOnIntegerOverflow=on  InputSameDT=on
  Switch : Switch  Threshold=0.5  InputSameDT=on
  Unit Delay3 : UnitDelay  Orientation=left  SampleTime=Ts
  itail : Outport  InitialOutput=0
  wires:
  1/1 -> Discrete-Time Integrator/1
  Discrete-Time Integrator/1 -> Look-Up Table/1
  Look-Up Table/1 -> Product/1
  Product/1 -> itail/1
  Switch/1 -> Unit Delay3/1, Product/2
  Unit Delay3/1 -> Switch/3
  Iak/1 -> Switch/1
  switch/1 -> Discrete-Time Integrator/2, Switch/2

== system powerlib_models/Discrete/GTO-IGBT Bridge/Vf  ==
  status_GTO : Inport  Port=1  LatchInput=off
  Switch : Switch  Threshold=0.5  InputSameDT=on
  Unit Delay9 : UnitDelay  SampleTime=Ts
  Vf device : Constant  Value=Vf*ones(nb_switch,1)
  Vf diode : Constant  Value=-Vfd*ones(nb_switch,1)
  Vf : Outport  InitialOutput=[0]
  wires:
  Unit Delay9/1 -> Vf/1
  status_GTO/1 -> Switch/2
  Switch/1 -> Unit Delay9/1
  Vf diode/1 -> Switch/3
  Vf device/1 -> Switch/1

== system powerlib_models/Discrete/HTG/Discrete PID Controller ==
  note: Discrete PID Controller
  note: Pierre Giroux, Gilbert Sybille
      | Power System Simulation Laboratory
      | IREQ, Hydro-Quebc
  Error : Inport  Port=1  LatchInput=off
  "Derivative " : DiscreteTransferFcn  Numerator=[2 -2]  Denominator=[Ts+2*TcD Ts-2*TcD]  SampleTime=Ts
  Discrete-Time Integrator : DiscreteIntegrator  InitialCondition=Init  SampleTime=Ts  LimitOutput=on  UpperSaturationLimit=UpperLimit  LowerSaturationLimit=LowerLimit  ICPrevOutput=DiscIntNeverNeededParam  ICPrevScaledInput=DiscIntNeverNeededParam
  Kp4 : Gain  Gain=Kp  SaturateOnIntegerOverflow=on
  Kp5 : Gain  Gain=Ki  SaturateOnIntegerOverflow=on
  Kp6 : Gain  Gain=Kd  SaturateOnIntegerOverflow=on
  Saturation2 : Saturate  UpperLimit=UpperLimit  LowerLimit=LowerLimit
  Sum6 : Sum  Inputs=+++  SaturateOnIntegerOverflow=on  InputSameDT=on
  Out : Outport  InitialOutput=0
  wires:
  Error/1 -> Kp4/1, Kp5/1, Kp6/1
  Sum6/1 -> Saturation2/1
  Kp5/1 -> Discrete-Time Integrator/1
  Kp6/1 -> "Derivative "/1
  Kp4/1 -> Sum6/1
  Discrete-Time Integrator/1 -> Sum6/2
  "Derivative "/1 -> Sum6/3
  Saturation2/1 -> Out/1

== system powerlib_models/Discrete/HTG/servo-motor ==
  regulator's output : Inport  Port=1  LatchInput=off
  Sum4 : Sum  Inputs=+-  SaturateOnIntegerOverflow=on  InputSameDT=on
  position : DiscreteIntegrator  InitialCondition=go  SampleTime=Ts  LimitOutput=on  UpperSaturationLimit=gmax  LowerSaturationLimit=gmin  ICPrevOutput=DiscIntNeverNeededParam  ICPrevScaledInput=DiscIntNeverNeededParam
  servo-motor : Subsystem
  speed limit : Saturate  UpperLimit=vgmax  LowerLimit=vgmin
  gate opening : Outport  InitialOutput=0
  wires:
  position/1 -> Sum4/2, gate opening/1
  speed limit/1 -> position/1
  servo-motor/1(Out) -> speed limit/1
  Sum4/1 -> servo-motor/1(In)
  regulator's output/1 -> Sum4/1

== system powerlib_models/Discrete/HTG/turbine ==
  dw : Inport  Port=1  LatchInput=off
  gate opening : Inport  Port=2  LatchInput=off
  Constant : Constant  Orientation=left
  Fcn : Fcn  Expr=(u(2)/u(1))^2
  Gain2 : Gain  Orientation=left  Gain=1/tw  SaturateOnIntegerOverflow=on
  Mux : Mux  Inputs=2
  Product : Product  SaturateOnIntegerOverflow=on  InputSameDT=on
  Sum2 : Sum  Inputs=-+  SaturateOnIntegerOverflow=on  InputSameDT=on
  Sum3 : Sum  Orientation=left  Inputs=-+  SaturateOnIntegerOverflow=on  InputSameDT=on
  beta : Gain  Gain=beta  SaturateOnIntegerOverflow=on
  position : DiscreteIntegrator  Orientation=left  InitialCondition=po  SampleTime=Ts  UpperSaturationLimit=0  LowerSaturationLimit=0  ICPrevOutput=DiscIntNeverNeededParam  ICPrevScaledInput=DiscIntNeverNeededParam
  turbine gain : Gain  Gain=1/(gmax-gmin)  SaturateOnIntegerOverflow=on
  Pm : Outport  InitialOutput=0
  wires:
  turbine gain/1 -> Mux/1
  gate opening/1 -> turbine gain/1
  Mux/1 -> Fcn/1
  Fcn/1 -> Sum2/2
  Constant/1 -> Sum3/2
  Product/1 -> Pm/1
  Sum3/1 -> Gain2/1
  Gain2/1 -> position/1
  Sum2/1 -> Sum3/1, Product/1
  beta/1 -> Sum2/1
  dw/1 -> beta/1
  position/1 -> Product/2, Mux/2

== system powerlib_models/Discrete/MBPSS/Discrete Lead-Lag1 ==
  In1 : Inport  Port=1  LatchInput=off
  Discrete State-Space : DiscreteStateSpace  A=Ad  B=Bd  C=Cd  D=Dd  SampleTime=Ts
  Out1 : Outport
  wires:
  Discrete State-Space/1 -> Out1/1
  In1/1 -> Discrete State-Space/1

== system powerlib_models/Discrete/MBPSS/Discrete Lead-Lag2 ==
  In1 : Inport  Port=1  LatchInput=off
  Discrete State-Space : DiscreteStateSpace  A=Ad  B=Bd  C=Cd  D=Dd  SampleTime=Ts
  Out1 : Outport
  wires:
  In1/1 -> Discrete State-Space/1
  Discrete State-Space/1 -> Out1/1

== system powerlib_models/Discrete/MBPSS/Discrete Lead-Lag3 ==
  In1 : Inport  Port=1  LatchInput=off
  Discrete State-Space : DiscreteStateSpace  A=Ad  B=Bd  C=Cd  D=Dd  SampleTime=Ts
  Out1 : Outport
  wires:
  In1/1 -> Discrete State-Space/1
  Discrete State-Space/1 -> Out1/1

== system powerlib_models/Discrete/MBPSS/Discrete Lead-Lag4 ==
  In1 : Inport  Port=1  LatchInput=off
  Discrete State-Space : DiscreteStateSpace  A=Ad  B=Bd  C=Cd  D=Dd  SampleTime=Ts
  Out1 : Outport
  wires:
  Discrete State-Space/1 -> Out1/1
  In1/1 -> Discrete State-Space/1

== system powerlib_models/Discrete/MBPSS/Discrete Lead-Lag5 ==
  In1 : Inport  Port=1  LatchInput=off
  Discrete State-Space : DiscreteStateSpace  A=Ad  B=Bd  C=Cd  D=Dd  SampleTime=Ts
  Out1 : Outport
  wires:
  Discrete State-Space/1 -> Out1/1
  In1/1 -> Discrete State-Space/1

== system powerlib_models/Discrete/MBPSS/Discrete Lead-Lag6 ==
  In1 : Inport  Port=1  LatchInput=off
  Discrete State-Space : DiscreteStateSpace  A=Ad  B=Bd  C=Cd  D=Dd  SampleTime=Ts
  Out1 : Outport
  wires:
  In1/1 -> Discrete State-Space/1
  Discrete State-Space/1 -> Out1/1

== system powerlib_models/Discrete/MBPSS/HF speed sensor ==
  In : Inport  Port=1  LatchInput=off
  Discrete State-Space : DiscreteStateSpace  A=Ad  B=Bd  C=Cd  D=Dd  SampleTime=Ts
  Out : Outport
  wires:
  Discrete State-Space/1 -> Out/1
  In/1 -> Discrete State-Space/1

== system powerlib_models/Discrete/MBPSS/LF and IF speed sensor ==
  In : Inport  Port=1  LatchInput=off
  Discrete State-Space : DiscreteStateSpace  A=Ad  B=Bd  C=Cd  D=Dd  SampleTime=Ts
  Out : Outport
  wires:
  Discrete State-Space/1 -> Out/1
  In/1 -> Discrete State-Space/1

== system powerlib_models/Discrete/MBPSS/Transfer function for detailed model (HF) ==
  On : Inport  Port=1  LatchInput=off
  "HFpos " : Inport  Port=2  LatchInput=off
  "HFneg " : Inport  Port=3  LatchInput=off
  Switch1 : Switch  Threshold=0.5  InputSameDT=on
  Switch2 : Switch  Threshold=0.5  InputSameDT=on
  Transfer functions for detailed stabilizer : Subsystem  TreatAsAtomicUnit=on
  Transfer functions for detailed stabilizer1 : Subsystem  TreatAsAtomicUnit=on
  HFpos : Outport
  LFneg : Outport  Port=2
  wires:
  On/1 -> Transfer functions for detailed stabilizer1/Enable, Switch2/2, Switch1/2, Transfer functions for detailed stabilizer/Enable
  Transfer functions for detailed stabilizer1/1(Out1) -> Switch2/1
  Switch2/1 -> LFneg/1
  "HFneg "/1 -> Transfer functions for detailed stabilizer1/1(In1), Switch2/3
  Switch1/1 -> HFpos/1
  "HFpos "/1 -> Switch1/3, Transfer functions for detailed stabilizer/1(In1)
  Transfer functions for detailed stabilizer/1(Out1) -> Switch1/1

== system powerlib_models/Discrete/MBPSS/Transfer function for detailed model (IF) ==
  On : Inport  Port=1  LatchInput=off
  "IFpos " : Inport  Port=2  LatchInput=off
  "IFneg " : Inport  Port=3  LatchInput=off
  Switch1 : Switch  Threshold=0.5  InputSameDT=on
  Switch2 : Switch  Threshold=0.5  InputSameDT=on
  Transfer functions for detailed stabilizer : Subsystem  TreatAsAtomicUnit=on
  Transfer functions for detailed stabilizer1 : Subsystem  TreatAsAtomicUnit=on
  IFpos : Outport
  IFneg : Outport  Port=2
  wires:
  Transfer functions for detailed stabilizer/1(Out1) -> Switch1/1
  "IFpos "/1 -> Transfer functions for detailed stabilizer/1(In1), Switch1/3
  Switch1/1 -> IFpos/1
  "IFneg "/1 -> Switch2/3, Transfer functions for detailed stabilizer1/1(In1)
  Switch2/1 -> IFneg/1
  Transfer functions for detailed stabilizer1/1(Out1) -> Switch2/1
  On/1 -> Transfer functions for detailed stabilizer/Enable, Switch1/2, Switch2/2, Transfer functions for detailed stabilizer1/Enable

== system powerlib_models/Discrete/MBPSS/Transfer function for detailed model (LF) ==
  On : Inport  Port=1  LatchInput=off
  "LFpos " : Inport  Port=2  LatchInput=off
  "LFneg " : Inport  Port=3  LatchInput=off
  Switch1 : Switch  Threshold=0.5  InputSameDT=on
  Switch2 : Switch  Threshold=0.5  InputSameDT=on
  Transfer functions for detailed stabilizer : Subsystem  TreatAsAtomicUnit=on
  Transfer functions for detailed stabilizer1 : Subsystem  TreatAsAtomicUnit=on
  LFpos : Outport
  LFneg : Outport  Port=2
  wires:
  On/1 -> Transfer functions for detailed stabilizer1/Enable, Switch2/2, Switch1/2, Transfer functions for detailed stabilizer/Enable
  Transfer functions for detailed stabilizer1/1(Out1) -> Switch2/1
  Switch2/1 -> LFneg/1
  "LFneg "/1 -> Transfer functions for detailed stabilizer1/1(In1), Switch2/3
  Switch1/1 -> LFpos/1
  "LFpos "/1 -> Switch1/3, Transfer functions for detailed stabilizer/1(In1)
  Transfer functions for detailed stabilizer/1(Out1) -> Switch1/1

== system powerlib_models/Discrete/PM_synchronous_machine/abc2qd ==
  note: This subsystem converts Vab and Vbc to Vd,Vq. The sine and cosine com-
      | puted here are sent to the inverse transformation subsystem dq2abc.
  Vab,Vbc : Inport  Port=1  LatchInput=off
  the : Inport  Port=2  LatchInput=off
  Elementary Math : ElementaryMath
  Elementary Math1 : ElementaryMath  Operator=cos
  Fcn2 : Fcn  Expr=(u[4]*(2*u[1]+u[2]) + (sqrt3*u[2]*u[3])) * one_third
  Fcn3 : Fcn  Expr=(u[3]*(2*u[1]+u[2]) + (-sqrt3*u[2]*u[4])) * one_third
  Mux1 : Mux  Inputs=[ 2 2 ]
  Mux2 : Mux  Inputs=2
  Mux3 : Mux  Inputs=2
  s,c : Outport  InitialOutput=0
  vq,vd : Outport  Port=2  InitialOutput=0
  wires:
  Mux1/1 -> Fcn2/1, Fcn3/1
  Mux3/1 -> s,c/1, Mux1/2
  Fcn2/1 -> Mux2/1
  Fcn3/1 -> Mux2/2
  Mux2/1 -> vq,vd/1
  Vab,Vbc/1 -> Mux1/1
  Elementary Math/1 -> Mux3/1
  Elementary Math1/1 -> Mux3/2
  the/1 -> Elementary Math/1, Elementary Math1/1

== system powerlib_models/Discrete/PM_synchronous_machine/iq,id ==
  vq,vd : Inport  Port=1  LatchInput=off
  we : Inport  Port=2  LatchInput=off
  Demux : Demux  Outputs=2
  Mux : Mux  Inputs=2
  id : Subsystem
  iq : Subsystem
  iq,id : Outport  InitialOutput=0
  wires:
  we/1 -> iq/2(we), id/2(we)
  id/1(id) -> Mux/2, iq/3(id)
  iq/1(iq) -> Mux/1, id/1(iq)
  Demux/2 -> id/3(vd)
  Demux/1 -> iq/1(vq)
  vq,vd/1 -> Demux/1
  Mux/1 -> iq,id/1

== system powerlib_models/Discrete/PM_synchronous_machine/qd2abc ==
  s,c : Inport  Port=1  LatchInput=off
  iq,id : Inport  Port=2  LatchInput=off
  Fcn : Fcn  Expr=u[3]*u[2] + u[4]*u[1]
  Fcn1 : Fcn  Expr=(u[2]*(-u[3]-sqrt3*u[4]) + u[1]*(sqrt3*u[3]-u[4]))*0.5
  Mux : Mux  Inputs=[2,2]
  Mux2 : Mux  Inputs=3
  Sum : Sum  Orientation=down  Inputs=--  SaturateOnIntegerOverflow=on  InputSameDT=on
  is : Outport  InitialOutput=0
  wires:
  Mux/1 -> Fcn/1, Fcn1/1
  s,c/1 -> Mux/1
  iq,id/1 -> Mux/2
  Sum/1 -> Mux2/3
  Fcn/1 -> Mux2/1, Sum/2
  Fcn1/1 -> Mux2/2, Sum/1
  Mux2/1 -> is/1

== system powerlib_models/Discrete/PSS/Lead-Lag #1 ==
  In1 : Inport  Port=1  LatchInput=off
  Discrete State-Space : DiscreteStateSpace  A=Ad  B=Bd  C=Cd  D=Dd  X0=x0d  SampleTime=Ts
  Out1 : Outport
  wires:
  Discrete State-Space/1 -> Out1/1
  In1/1 -> Discrete State-Space/1

== system powerlib_models/Discrete/PSS/Lead-Lag #2 ==
  In1 : Inport  Port=1  LatchInput=off
  Discrete State-Space : DiscreteStateSpace  A=Ad  B=Bd  C=Cd  D=Dd  X0=x0d  SampleTime=Ts
  Out1 : Outport
  wires:
  Discrete State-Space/1 -> Out1/1
  In1/1 -> Discrete State-Space/1

== system powerlib_models/Discrete/PSS/Sensor  ==
  In : Inport  Port=1  LatchInput=off
  Discrete State-Space : DiscreteStateSpace  A=Ad  B=Bd  C=Cd  D=Dd  X0=x0d  SampleTime=Ts
  Out : Outport  InitialOutput=0
  wires:
  Discrete State-Space/1 -> Out/1
  In/1 -> Discrete State-Space/1

== system powerlib_models/Discrete/PSS/Wash-out  ==
  In : Inport  Port=1  LatchInput=off
  Discrete State-Space : DiscreteStateSpace  A=Ad  B=Bd  C=Cd  D=Dd  X0=x0d  SampleTime=Ts
  Out : Outport  InitialOutput=0
  wires:
  Discrete State-Space/1 -> Out/1
  In/1 -> Discrete State-Space/1

== system powerlib_models/Discrete/SSM_mechanics/Predict ==
  I : Inport  Port=1  LatchInput=off
  1\Llr4 : Gain  Gain=2  SaturateOnIntegerOverflow=on
  Sum5 : Sum  Inputs=+-  SaturateOnIntegerOverflow=on  InputSameDT=on
  Unit Delay2 : UnitDelay  X0=dwo  SampleTime=Ts
  O : Outport
  wires:
  1\Llr4/1 -> Sum5/1
  Unit Delay2/1 -> Sum5/2
  I/1 -> Unit Delay2/1, 1\Llr4/1
  Sum5/1 -> O/1

== system powerlib_models/Discrete/Three-Level Bridge/2-level GTO-IGBT Bridge  Logic (modified) ==
  note: Note 3: See Sw3 logic
  note: Diode Logic :
      | 1) Diodes are blocked when complementary GTOs are switched on
  v : Inport  Port=1  LatchInput=off
  g : Inport  Port=2  LatchInput=off
  Block12 : Inport  Port=3  LatchInput=off
  Trig12 : Inport  Port=4  LatchInput=off
  Data Type  Conversion2 : DataTypeConversion  OutDataTypeMode=double  SaturateOnIntegerOverflow=on  RndMeth=Zero
  Data Type  Conversion4 : DataTypeConversion  OutDataTypeMode=boolean  SaturateOnIntegerOverflow=on  RndMeth=Zero
  Demux1 : Demux  Outputs=[nb_arm nb_arm]
  Diode Logic : Subsystem
  GTO Logic : Subsystem
  G_D : Logic  Operator=OR
  G_D2 : Logic  Operator=NOT
  G_D3 : Logic  Operator=OR
  G_D4 : Logic  Operator=OR
  Gain : Gain  Orientation=up  Gain=-1  SaturateOnIntegerOverflow=on
  Gain1 : Gain  Gain=2  SaturateOnIntegerOverflow=on
  Note 3 : Logic
  Select_Block3 : Selector  Elements=Block3Elements  InputPortWidth=nb_switch
  Select_Vsw : Selector  Elements=VswElements  InputPortWidth=nb_arm*3
  Unit Delay3 : UnitDelay  SampleTime=Ts
  Unit Delay9 : UnitDelay  SampleTime=Ts
  "Vf " : Subsystem
  status : Outport
  Vf : Outport  Port=2
  Block3 : Outport  Port=3
  status_GTO : Outport  Port=4
  wires:
  G_D3/1 -> Block3/1
  Gain1/1 -> Unit Delay9/1
  G_D2/1 -> Note 3/2
  Block12/1 -> G_D2/1
  Diode Logic/1(status) -> Note 3/1
  Diode Logic/2(block) -> Select_Block3/1
  Gain/1 -> Diode Logic/1(Vak)
  v/1 -> Select_Vsw/1
  "Vf "/1(Vf) -> Gain1/1
  GTO Logic/1(status) -> G_D/2, Diode Logic/2(G), "Vf "/1(status_GTO), status_GTO/1
  g/1 -> Data Type  Conversion4/1
  Data Type  Conversion4/1 -> GTO Logic/2(G)
  Unit Delay3/1 -> status/1
  G_D/1 -> Data Type  Conversion2/1
  Data Type  Conversion2/1 -> Unit Delay3/1
  Unit Delay9/1 -> Vf/1
  G_D4/1 -> G_D/1
  Note 3/1 -> G_D4/1
  Trig12/1 -> G_D4/2
  Select_Vsw/1 -> Gain/1, GTO Logic/1(Vak)
  Select_Block3/1 -> Demux1/1
  Demux1/1 -> G_D3/1
  Demux1/2 -> G_D3/2

== system powerlib_models/Discrete/Three-Level Bridge/Input ==
  note: This block is required when the "pulses" input is not connected
  In : Inport  Port=1  LatchInput=off
  Constant : Constant
  require : Logic  OutDataTypeMode=Specify via dialog  LogicDataType=float('double')
  Out : Outport
  wires:
  Constant/1 -> require/2
  In/1 -> require/1
  require/1 -> Out/1

== system powerlib_models/Discrete/Three-Level Bridge/SubSystem ==
  note: D5, D6 : Clamping diodes
  note: - Vdc ------------
  note: N ----
  note: -[Sw3]-----
  note: |
      | |
      | |
      | [Q1 - D1]
      | |
      | |
  note: |
      | |
      | [Q2 - D2]
      | |
      | |
  note: |
      | |
      | [Q3 - D3]
      | |
      | |
  note: |
      | |
      | [Q4 - D4]
      | |
      | |
      | |
  note: -------[D5]-->-------
  note: -----<-[D6]---------
  note: ------------ A
  note: |
      | |
      | |
      | |
      | |
      | |
      | |
      | |
      | |
      | |
      | |
  note: N ----------
  note: - Vdc--------------------------
  note: + Vdc --------------------------
  note: ---------- A
  note: + Vdc ------------
  note: |
      | |
      | |
      | |
      | |
      | [Sw1]
      | |
      | |
      | |
      | |
  note: |
      | |
      | |
      | |
      | |
      | [Sw2]
      | |
      | |
      | |
      | |
  note: <======>
  note: (or B or C)
  note: (or B or C)

== system powerlib_models/Discrete/Three-Level Bridge/Sw3 (clamping diode) Logic ==
  note: Note 3: Diodes D1,D2,D3 and D4 are blocked for one step when diode 5 or 6 (Sw3) start conducting
  note: Note 4: When no pulses are sent to the valves:
      | trig (one time step) diodes D1 and D2 when diode D6 stop conducting or when Q3+Q4 stop conducting
      | or trig (one time step) diodes D3 and D4 when diode D5 stop conducting or when Q1+Q2 stop conducting.
  V_Sw123 : Inport  Port=1  LatchInput=off
  Pulses : Inport  Port=2  LatchInput=off
  Block3 : Inport  Port=3  LatchInput=off
  Status_GTO : Inport  Port=4  LatchInput=off
  0 2 : Constant  Value=0
  1 : Logic
  2 : Logic  Operator=NOT
  3 : Logic  Operator=OR
  4 : Logic
  5 : Logic
  6 : Logic  Operator=NOT
  Data Type  Conversion1 : DataTypeConversion  OutDataTypeMode=boolean  SaturateOnIntegerOverflow=on  RndMeth=Zero
  Data Type  Conversion2 : DataTypeConversion  OutDataTypeMode=double  SaturateOnIntegerOverflow=on  RndMeth=Zero
  Data Type  Conversion4 : DataTypeConversion  OutDataTypeMode=boolean  SaturateOnIntegerOverflow=on  RndMeth=Zero
  Demux : Demux  Outputs=[nb_arm nb_arm nb_arm nb_arm]
  Logical Operator : Logic
  Logical Operator1 : Logic
  Mux1 : Mux  Inputs=[nb_arm nb_arm]
  Note 3 : Subsystem
  Note 4 : Subsystem
  Select_Pulses : Selector  Elements=PulseElements  InputPortWidth=nb_arm*4
  Select_Vsw3 : Selector  Elements=Vsw3Elements  InputPortWidth=nb_arm*3
  Select_g12a : Selector  Elements=g12Elements  InputPortWidth=nb_arm*2
  Select_g12b : Selector  Elements=g12Elements  InputPortWidth=nb_arm*2
  Unit Delay1 : UnitDelay  SampleTime=Ts
  Unit Delay3 : UnitDelay  SampleTime=Ts
  Vf Computation for Sw3 : Subsystem
  b6 : RelationalOperator  Operator=<  InputSameDT=on
  Status : Outport
  Vf : Outport  Port=2
  g12 : Outport  Port=3
  Block12 : Outport  Port=4
  Trig12 : Outport  Port=5
  wires:
  Select_g12b/1 -> Trig12/1
  Select_g12a/1 -> g12/1
  Logical Operator/1 -> Mux1/1
  Select_Vsw3/1 -> b6/1
  5/1 -> Note 3/1(G), Data Type  Conversion2/1
  Note 3/1(Block.D) -> Block12/1
  Block3/1 -> 6/1
  Unit Delay3/1 -> Status/1
  2/1 -> 4/2
  V_Sw123/1 -> Select_Vsw3/1
  0 2/1 -> b6/2
  Pulses/1 -> Select_Pulses/1
  Mux1/1 -> Select_g12a/1
  Vf Computation for Sw3/1(Vf) -> Unit Delay1/1
  Unit Delay1/1 -> Vf/1
  Data Type  Conversion4/1 -> Demux/1, Note 4/1(pulses)
  Demux/1 -> Logical Operator/1  "Q1"
  Demux/2 -> Logical Operator/2, 1/1  "Q2"
  Demux/3 -> 4/1, Logical Operator1/1  "Q3"
  Demux/4 -> Logical Operator1/2  "Q4"
  Logical Operator1/1 -> Mux1/2
  b6/1 -> Data Type  Conversion1/1
  Data Type  Conversion1/1 -> 1/2, 2/1
  4/1 -> 3/2, Note 4/3(D6_On)  "D6_On"
  1/1 -> 3/1, Vf Computation for Sw3/1(D5_On), Note 4/2(D5_On)  "D5_On"
  3/1 -> 5/1
  6/1 -> 5/2
  Data Type  Conversion2/1 -> Unit Delay3/1
  Note 4/1(Trig12) -> Select_g12b/1
  Select_Pulses/1 -> Data Type  Conversion4/1
  Status_GTO/1 -> Note 4/4(Status_GTO)

== system powerlib_models/Discrete/asynchronous_machine/Mutual fluxes ==
  phiqr,phidr : Inport  Port=1  LatchInput=off
  phiqs,phids : Inport  Port=2  LatchInput=off
  1\Llr : Gain  Gain=1/Llr  SaturateOnIntegerOverflow=on
  1\Llr1 : Gain  Gain=Laq  SaturateOnIntegerOverflow=on
  1\Llr2 : Gain  Gain=Lad  SaturateOnIntegerOverflow=on
  1\Lls : Gain  Gain=1/Lls  SaturateOnIntegerOverflow=on
  Demux1 : Demux  Outputs=2
  Demux2 : Demux  Outputs=2
  Mux3 : Mux  Inputs=2
  Sum : Sum  Inputs=|++  SaturateOnIntegerOverflow=on  InputSameDT=on
  Sum1 : Sum  Inputs=++|  SaturateOnIntegerOverflow=on  InputSameDT=on
  phimq,phimd : Outport
  wires:
  Mux3/1 -> phimq,phimd/1
  1\Llr2/1 -> Mux3/2
  1\Llr1/1 -> Mux3/1
  Demux1/2 -> Sum1/1
  Demux2/2 -> Sum1/2
  Demux2/1 -> Sum/2
  1\Lls/1 -> Demux2/1
  Sum/1 -> 1\Llr1/1
  Demux1/1 -> Sum/1
  1\Llr/1 -> Demux1/1
  phiqr,phidr/1 -> 1\Llr/1
  phiqs,phids/1 -> 1\Lls/1
  Sum1/1 -> 1\Llr2/1
